simulink model "trial1"  (R2021a)
settings: Solver=VariableStepAuto  StartTime=0.0  StopTime=10  RelTol=1e-3
libraries: slpidlib x4, robotmobilelib x1
settings Model: Creator=templ  LastModifiedBy=templ

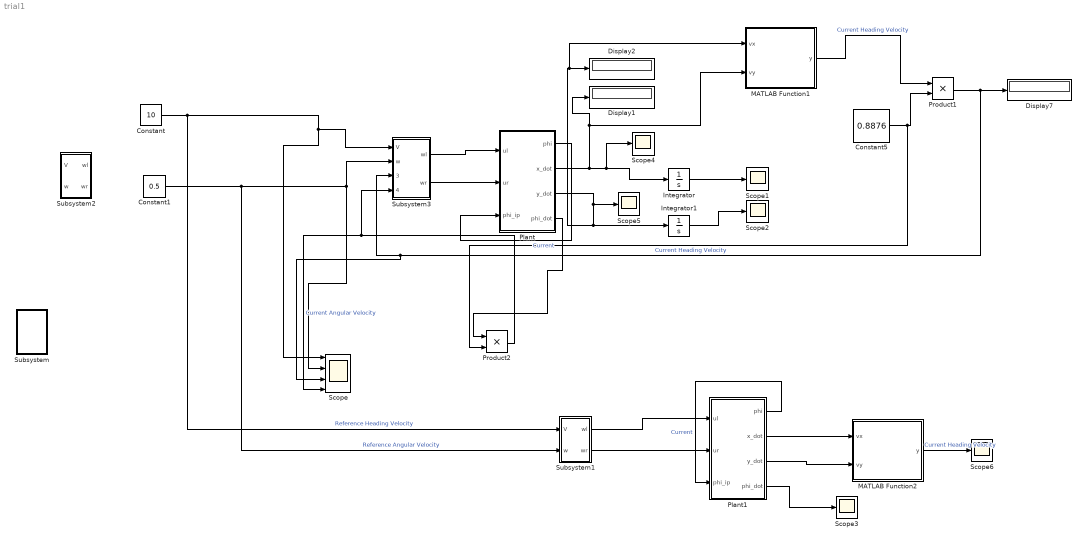
== system trial1 ==
  Constant : Constant  Value=10
  Constant1 : Constant  Value=0.5
  Constant5 : Constant  Value=0.8876
  Display1 : Display
  Display2 : Display
  Display7 : Display
  Integrator : Integrator
  Integrator1 : Integrator
  MATLAB Function1 : MATLAB Function  TreatAsAtomicUnit=on
  MATLAB Function2 : MATLAB Function  TreatAsAtomicUnit=on
  Plant : Subsystem
  Plant1 : Subsystem
  Product1 : Product
  Product2 : Product
  Scope : Scope  NumInputPorts=4
  Scope{1..6} (6 alike) : Scope
  Subsystem : Subsystem
  Subsystem1 : Subsystem
  Subsystem2 : Subsystem
  Subsystem3 : Subsystem
  wires:
  Plant/1(phi) -> Plant/3(phi_ip)  "Current"
  Plant/2(x_dot) -> MATLAB Function1/2(vy), Display1/1, Scope4/1, Integrator/1
  Plant/3(y_dot) -> Scope5/1, Integrator1/1, MATLAB Function1/1(vx), Display2/1
  Integrator/1 -> Scope1/1
  Integrator1/1 -> Scope2/1
  Plant/4(phi_dot) -> Product2/1
  MATLAB Function1/1(y) -> Product1/1  "Current Heading Velocity"
  Constant5/1 -> Product2/2, Product1/2
  Constant/1 -> Subsystem1/1(V), Scope/1, Subsystem3/1(V)  "Reference Heading Velocity"
  Constant1/1 -> Subsystem1/2(w), Subsystem3/2(w), Scope/2  "Reference Angular Velocity"
  Product1/1 -> Scope/3, Subsystem3/3(V_current), Display7/1  "Current Heading Velocity"
  Subsystem3/1(wl) -> Plant/1(ul)
  Subsystem3/2(wr) -> Plant/2(ur)
  Product2/1 -> Scope/4, Subsystem3/4(w_current)  "Current Angular Velocity"
  Plant1/1(phi) -> Plant1/3(phi_ip)  "Current"
  Plant1/2(x_dot) -> MATLAB Function2/1(vx)
  Plant1/3(y_dot) -> MATLAB Function2/2(vy)
  Plant1/4(phi_dot) -> Scope3/1
  MATLAB Function2/1(y) -> Scope6/1  "Current Heading Velocity"
  Subsystem1/1(wl) -> Plant1/1(ul)
  Subsystem1/2(wr) -> Plant1/2(ur)

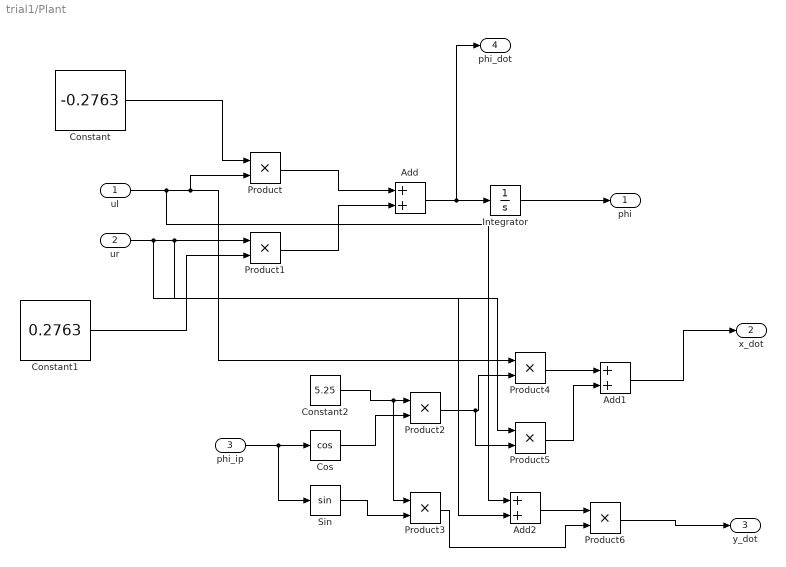
== system trial1/Plant ==
  ul : Inport
  ur : Inport  Port=2
  phi_ip : Inport  Port=3
  Add : Sum
  Add1 : Sum
  Add2 : Sum
  Constant : Constant  Value=-0.2763
  Constant1 : Constant  Value=0.2763
  Constant2 : Constant  Value=5.25
  Cos : Trigonometry  Operator=cos
  Integrator : Integrator
  Product{,1..6} (7 alike) : Product
  Sin : Trigonometry
  phi : Outport
  x_dot : Outport  Port=2
  y_dot : Outport  Port=3
  phi_dot : Outport  Port=4
  wires:
  ur/1 -> Add2/2, Product5/1, Product1/1
  Product/1 -> Add/1
  Integrator/1 -> phi/1
  Product1/1 -> Add/2
  Constant1/1 -> Product1/2
  Add/1 -> phi_dot/1, Integrator/1
  ul/1 -> Add2/1, Product4/1, Product/2
  Constant/1 -> Product/1
  phi_ip/1 -> Sin/1, Cos/1
  Cos/1 -> Product2/2
  Constant2/1 -> Product3/1, Product2/1
  Sin/1 -> Product3/2
  Product2/1 -> Product5/2, Product4/2
  Product4/1 -> Add1/1
  Product5/1 -> Add1/2
  Add1/1 -> x_dot/1
  Add2/1 -> Product6/1
  Product3/1 -> Product6/2
  Product6/1 -> y_dot/1

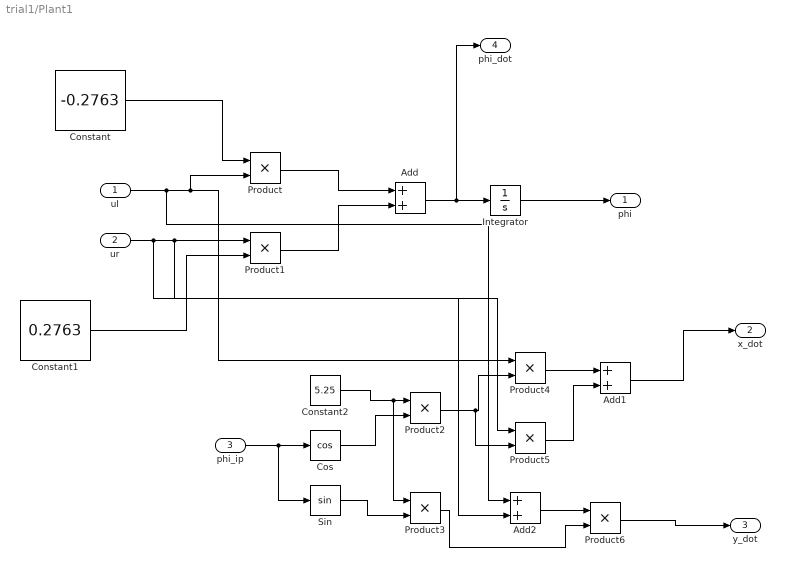
== system trial1/Plant1 ==
  ul : Inport
  ur : Inport  Port=2
  phi_ip : Inport  Port=3
  Add : Sum
  Add1 : Sum
  Add2 : Sum
  Constant : Constant  Value=-0.2763
  Constant1 : Constant  Value=0.2763
  Constant2 : Constant  Value=5.25
  Cos : Trigonometry  Operator=cos
  Integrator : Integrator
  Product{,1..6} (7 alike) : Product
  Sin : Trigonometry
  phi : Outport
  x_dot : Outport  Port=2
  y_dot : Outport  Port=3
  phi_dot : Outport  Port=4
  wires:
  ur/1 -> Add2/2, Product5/1, Product1/1
  Product/1 -> Add/1
  Integrator/1 -> phi/1
  Product1/1 -> Add/2
  Constant1/1 -> Product1/2
  Add/1 -> phi_dot/1, Integrator/1
  ul/1 -> Add2/1, Product4/1, Product/2
  Constant/1 -> Product/1
  phi_ip/1 -> Sin/1, Cos/1
  Cos/1 -> Product2/2
  Constant2/1 -> Product3/1, Product2/1
  Sin/1 -> Product3/2
  Product2/1 -> Product5/2, Product4/2
  Product4/1 -> Add1/1
  Product5/1 -> Add1/2
  Add1/1 -> x_dot/1
  Add2/1 -> Product6/1
  Product3/1 -> Product6/2
  Product6/1 -> y_dot/1

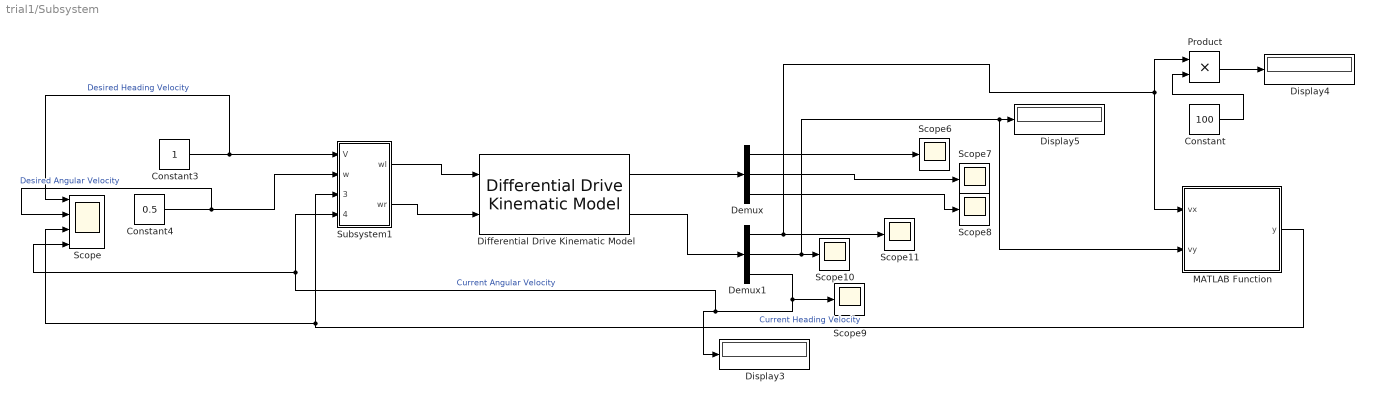
== system trial1/Subsystem ==
  Constant : Constant  Value=100
  Constant3 : Constant
  Constant4 : Constant  Value=0.5
  Demux : Demux  Outputs=3
  Demux1 : Demux  Outputs=3
  Differential Drive Kinematic Model : robotmobilelib/Differential Drive Kinematic Model  VehicleInputs=Wheel Speeds  WheelRadius=0.105  WheelSpeedRange=[-inf inf]  TrackWidth=0.05  InitialState=[0; 0; 0]  SimulateUsing=Interpreted execution
      settings: SourceProductBaseCode=RO
  Display3 : Display
  Display4 : Display
  Display5 : Display
  MATLAB Function : MATLAB Function  TreatAsAtomicUnit=on
  Product : Product
  Scope : Scope  NumInputPorts=4
  Scope{6..11} (6 alike) : Scope
  Subsystem1 : Subsystem
  wires:
  Demux1/2 -> MATLAB Function/2(vy), Display5/1, Scope10/1
  Differential Drive Kinematic Model/2 -> Demux1/1
  Constant3/1 -> Scope/1, Subsystem1/1(V)  "Desired Heading Velocity"
  MATLAB Function/1(y) -> Scope/3, Subsystem1/3(V_current)  "Current Heading Velocity"
  Demux1/1 -> MATLAB Function/1(vx), Product/1, Scope11/1
  Demux1/3 -> Scope/4, Subsystem1/4(w_current), Display3/1, Scope9/1  "Current Angular Velocity"
  Differential Drive Kinematic Model/1 -> Demux/1
  Demux/3 -> Scope8/1
  Constant4/1 -> Scope/2, Subsystem1/2(w)  "Desired Angular Velocity"
  Product/1 -> Display4/1
  Constant/1 -> Product/2
  Subsystem1/1(wl) -> Differential Drive Kinematic Model/1
  Subsystem1/2(wr) -> Differential Drive Kinematic Model/2
  Demux/2 -> Scope7/1
  Demux/1 -> Scope6/1

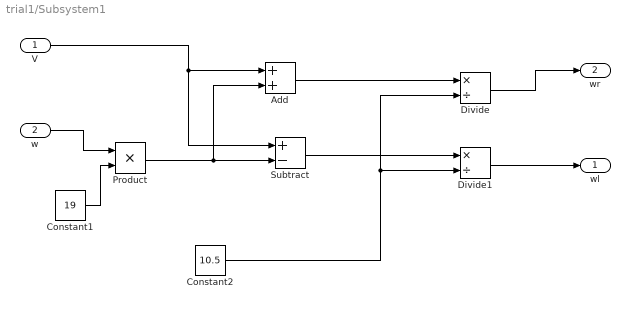
== system trial1/Subsystem1 ==
  V : Inport
  w : Inport  Port=2
  Add : Sum
  Constant1 : Constant  Value=19
  Constant2 : Constant  Value=10.5
  Divide : Product  Inputs=*/
  Divide1 : Product  Inputs=*/
  Product : Product
  Subtract : Sum  Inputs=+-
  wl : Outport
  wr : Outport  Port=2
  wires:
  V/1 -> Subtract/1, Add/1
  Add/1 -> Divide/1
  Constant2/1 -> Divide1/2, Divide/2
  Subtract/1 -> Divide1/1
  Product/1 -> Subtract/2, Add/2
  Divide1/1 -> wl/1
  Divide/1 -> wr/1
  Constant1/1 -> Product/2
  w/1 -> Product/1

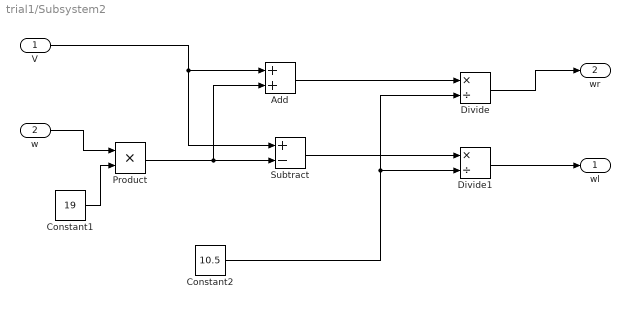
== system trial1/Subsystem2 ==
  V : Inport
  w : Inport  Port=2
  Add : Sum
  Constant1 : Constant  Value=19
  Constant2 : Constant  Value=10.5
  Divide : Product  Inputs=*/
  Divide1 : Product  Inputs=*/
  Product : Product
  Subtract : Sum  Inputs=+-
  wl : Outport
  wr : Outport  Port=2
  wires:
  V/1 -> Subtract/1, Add/1
  Add/1 -> Divide/1
  Constant2/1 -> Divide1/2, Divide/2
  Subtract/1 -> Divide1/1
  Product/1 -> Subtract/2, Add/2
  Divide1/1 -> wl/1
  Divide/1 -> wr/1
  Constant1/1 -> Product/2
  w/1 -> Product/1

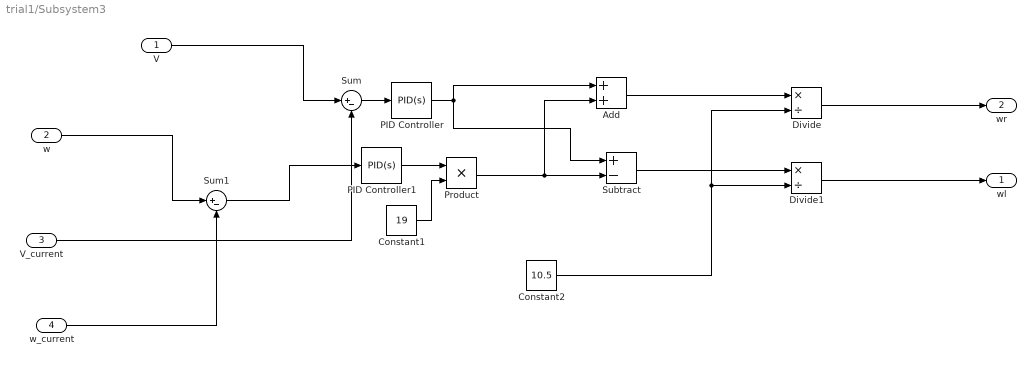
== system trial1/Subsystem3 ==
  V : Inport
  w : Inport  Port=2
  V_current : Inport  Port=3
  w_current : Inport  Port=4
  Add : Sum
  Constant1 : Constant  Value=19
  Constant2 : Constant  Value=10.5
  Divide : Product  Inputs=*/
  Divide1 : Product  Inputs=*/
  PID Controller : slpidlib/PID Controller  Controller=PID  Form=Parallel  TimeDomain=Continuous-time  UseExternalTs=off  SampleTime=-1  IntegratorMethod=Forward Euler  FilterMethod=Forward Euler  ControllerParametersSource=internal  P=10  I=1  D=5  UseFilter=on  N=100  TunerSelectOption=Transfer Function Based (PID Tuner App)  InitialConditionSource=internal  InitialConditionForIntegrator=0  InitialConditionForFilter=0  DifferentiatorICPrevScaledInput=0  ExternalReset=none  TrackingMode=off  Kt=1  LimitOutput=off  SatLimitsSource=internal  UpperSaturationLimit=inf  LowerSaturationLimit=-inf  LinearizeAsGain=on  AntiWindupMode=none  Kb=1  POutMin=[]  POutMax=[]  IOutMin=[]  IOutMax=[]  DOutMin=[]  DOutMax=[]  NOutMin=[]  NOutMax=[]  SumOutMin=[]  SumOutMax=[]  SaturationOutMin=[]  SaturationOutMax=[]  PParamMin=[]  PParamMax=[]  IParamMin=[]  IParamMax=[]  DParamMin=[]  DParamMax=[]  NParamMin=[]  NParamMax=[]  KbParamMin=[]  KbParamMax=[]  KtParamMin=[]  KtParamMax=[]  KbOutMin=[]  KbOutMax=[]  KtOutMin=[]  KtOutMax=[]  IntegratorOutMin=[]  IntegratorOutMax=[]  FilterOutMin=[]  FilterOutMax=[]  SumI1OutMin=[]  SumI1OutMax=[]  SumI2OutMin=[]  SumI2OutMax=[]  SumI3OutMin=[]  SumI3OutMax=[]  SumI4OutMin=[]  SumI4OutMax=[]  SumDOutMin=[]  SumDOutMax=[]  DifferentiatorOutMin=[]  DifferentiatorOutMax=[]  FilterDiffOutCoefMin=[]  FilterDiffOutCoefMax=[]  ReciprocalOutMin=[]  ReciprocalOutMax=[]  SumDenOutMin=[]  SumDenOutMax=[]  SumNumOutMin=[]  SumNumOutMax=[]  DivideOutMin=[]  DivideOutMax=[]  UdiffTsProdOutMin=[]  UdiffTsProdOutMax=[]  NTsProdOutMin=[]  NTsProdOutMax=[]  UintegralTsProdOutMin=[]  UintegralTsProdOutMax=[]  UngainTsProdOutMin=[]  UngainTsProdOutMax=[]  IntegratorContinuousStateAttributes=''  IntegratorStateMustResolveToSignalObject=off  IntegratorRTWStateStorageClass=Auto  FilterContinuousStateAttributes=''  FilterStateMustResolveToSignalObject=off  FilterRTWStateStorageClass=Auto  ParallelPVariant=InternalParameters  IdealPVariant=Disabled  IVariant=InternalParameters  DVariant=InternalParameters  IntegratorVariant=Continuous  SatVariant=Disabled  AWVariant=Passthrough  PCopyVariant=Disabled  TRVariant=Disabled  FdbkBlocksVariant=Forward  IdealPFdbkVariant=Disabled  SatFdbkVariant=Disabled  DerivativeFilterVariant=ContFilter  NVariant=InternalParameters  NCopyVariant=Disabled  FilterICVariant=InternalICsFilter  IntegratorICVariant=InternalICs  ExternalResetVariant=Disabled  TRSumVariant=Passthrough  SumFdbkVariant=Disabled  SumVariant=Sum_PID  TsampFilterVariant=InternalTs  TsampNgainVariant=Passthrough  TsampIntegralVariant=Passthrough  ExternalSaturationOutDataTypeStr=Inherit: Same as second input
  PID Controller1 : slpidlib/PID Controller  Controller=PID  Form=Parallel  TimeDomain=Continuous-time  UseExternalTs=off  SampleTime=-1  IntegratorMethod=Forward Euler  FilterMethod=Forward Euler  ControllerParametersSource=internal  P=10  I=1  D=5  UseFilter=on  N=100  TunerSelectOption=Transfer Function Based (PID Tuner App)  InitialConditionSource=internal  InitialConditionForIntegrator=0  InitialConditionForFilter=0  DifferentiatorICPrevScaledInput=0  ExternalReset=none  TrackingMode=off  Kt=1  LimitOutput=off  SatLimitsSource=internal  UpperSaturationLimit=inf  LowerSaturationLimit=-inf  LinearizeAsGain=on  AntiWindupMode=none  Kb=1  POutMin=[]  POutMax=[]  IOutMin=[]  IOutMax=[]  DOutMin=[]  DOutMax=[]  NOutMin=[]  NOutMax=[]  SumOutMin=[]  SumOutMax=[]  SaturationOutMin=[]  SaturationOutMax=[]  PParamMin=[]  PParamMax=[]  IParamMin=[]  IParamMax=[]  DParamMin=[]  DParamMax=[]  NParamMin=[]  NParamMax=[]  KbParamMin=[]  KbParamMax=[]  KtParamMin=[]  KtParamMax=[]  KbOutMin=[]  KbOutMax=[]  KtOutMin=[]  KtOutMax=[]  IntegratorOutMin=[]  IntegratorOutMax=[]  FilterOutMin=[]  FilterOutMax=[]  SumI1OutMin=[]  SumI1OutMax=[]  SumI2OutMin=[]  SumI2OutMax=[]  SumI3OutMin=[]  SumI3OutMax=[]  SumI4OutMin=[]  SumI4OutMax=[]  SumDOutMin=[]  SumDOutMax=[]  DifferentiatorOutMin=[]  DifferentiatorOutMax=[]  FilterDiffOutCoefMin=[]  FilterDiffOutCoefMax=[]  ReciprocalOutMin=[]  ReciprocalOutMax=[]  SumDenOutMin=[]  SumDenOutMax=[]  SumNumOutMin=[]  SumNumOutMax=[]  DivideOutMin=[]  DivideOutMax=[]  UdiffTsProdOutMin=[]  UdiffTsProdOutMax=[]  NTsProdOutMin=[]  NTsProdOutMax=[]  UintegralTsProdOutMin=[]  UintegralTsProdOutMax=[]  UngainTsProdOutMin=[]  UngainTsProdOutMax=[]  IntegratorContinuousStateAttributes=''  IntegratorStateMustResolveToSignalObject=off  IntegratorRTWStateStorageClass=Auto  FilterContinuousStateAttributes=''  FilterStateMustResolveToSignalObject=off  FilterRTWStateStorageClass=Auto  ParallelPVariant=InternalParameters  IdealPVariant=Disabled  IVariant=InternalParameters  DVariant=InternalParameters  IntegratorVariant=Continuous  SatVariant=Disabled  AWVariant=Passthrough  PCopyVariant=Disabled  TRVariant=Disabled  FdbkBlocksVariant=Forward  IdealPFdbkVariant=Disabled  SatFdbkVariant=Disabled  DerivativeFilterVariant=ContFilter  NVariant=InternalParameters  NCopyVariant=Disabled  FilterICVariant=InternalICsFilter  IntegratorICVariant=InternalICs  ExternalResetVariant=Disabled  TRSumVariant=Passthrough  SumFdbkVariant=Disabled  SumVariant=Sum_PID  TsampFilterVariant=InternalTs  TsampNgainVariant=Passthrough  TsampIntegralVariant=Passthrough  ExternalSaturationOutDataTypeStr=Inherit: Same as second input
  Product : Product
  Subtract : Sum  Inputs=+-
  Sum : Sum  Inputs=|+-
  Sum1 : Sum  Inputs=|+-
  wl : Outport
  wr : Outport  Port=2
  wires:
  V/1 -> Sum/1
  Add/1 -> Divide/1
  Constant2/1 -> Divide1/2, Divide/2
  Subtract/1 -> Divide1/1
  Product/1 -> Subtract/2, Add/2
  Constant1/1 -> Product/2
  w/1 -> Sum1/1
  V_current/1 -> Sum/2
  Sum/1 -> PID Controller/1
  w_current/1 -> Sum1/2
  Sum1/1 -> PID Controller1/1
  PID Controller/1 -> Subtract/1, Add/1
  PID Controller1/1 -> Product/1
  Divide/1 -> wr/1
  Divide1/1 -> wl/1

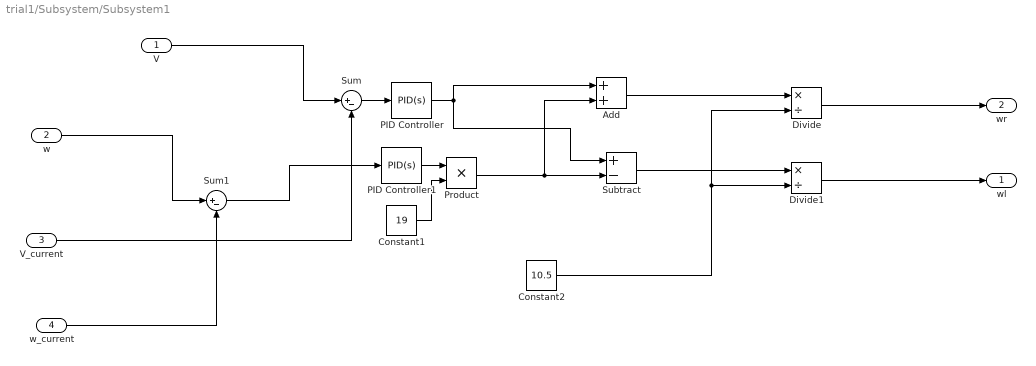
== system trial1/Subsystem/Subsystem1 ==
  V : Inport
  w : Inport  Port=2
  V_current : Inport  Port=3
  w_current : Inport  Port=4
  Add : Sum
  Constant1 : Constant  Value=19
  Constant2 : Constant  Value=10.5
  Divide : Product  Inputs=*/
  Divide1 : Product  Inputs=*/
  PID Controller : slpidlib/PID Controller  Controller=PID  Form=Parallel  TimeDomain=Continuous-time  UseExternalTs=off  SampleTime=-1  IntegratorMethod=Forward Euler  FilterMethod=Forward Euler  ControllerParametersSource=internal  P=-500  I=100  D=1  UseFilter=on  N=100  TunerSelectOption=Frequency Response Based  InitialConditionSource=internal  InitialConditionForIntegrator=0  InitialConditionForFilter=0  DifferentiatorICPrevScaledInput=0  ExternalReset=none  TrackingMode=off  Kt=1  LimitOutput=off  SatLimitsSource=internal  UpperSaturationLimit=inf  LowerSaturationLimit=-inf  LinearizeAsGain=on  AntiWindupMode=none  Kb=1  POutMin=[]  POutMax=[]  IOutMin=[]  IOutMax=[]  DOutMin=[]  DOutMax=[]  NOutMin=[]  NOutMax=[]  SumOutMin=[]  SumOutMax=[]  SaturationOutMin=[]  SaturationOutMax=[]  PParamMin=[]  PParamMax=[]  IParamMin=[]  IParamMax=[]  DParamMin=[]  DParamMax=[]  NParamMin=[]  NParamMax=[]  KbParamMin=[]  KbParamMax=[]  KtParamMin=[]  KtParamMax=[]  KbOutMin=[]  KbOutMax=[]  KtOutMin=[]  KtOutMax=[]  IntegratorOutMin=[]  IntegratorOutMax=[]  FilterOutMin=[]  FilterOutMax=[]  SumI1OutMin=[]  SumI1OutMax=[]  SumI2OutMin=[]  SumI2OutMax=[]  SumI3OutMin=[]  SumI3OutMax=[]  SumI4OutMin=[]  SumI4OutMax=[]  SumDOutMin=[]  SumDOutMax=[]  DifferentiatorOutMin=[]  DifferentiatorOutMax=[]  FilterDiffOutCoefMin=[]  FilterDiffOutCoefMax=[]  ReciprocalOutMin=[]  ReciprocalOutMax=[]  SumDenOutMin=[]  SumDenOutMax=[]  SumNumOutMin=[]  SumNumOutMax=[]  DivideOutMin=[]  DivideOutMax=[]  UdiffTsProdOutMin=[]  UdiffTsProdOutMax=[]  NTsProdOutMin=[]  NTsProdOutMax=[]  UintegralTsProdOutMin=[]  UintegralTsProdOutMax=[]  UngainTsProdOutMin=[]  UngainTsProdOutMax=[]  IntegratorContinuousStateAttributes=''  IntegratorStateMustResolveToSignalObject=off  IntegratorRTWStateStorageClass=Auto  FilterContinuousStateAttributes=''  FilterStateMustResolveToSignalObject=off  FilterRTWStateStorageClass=Auto  ParallelPVariant=InternalParameters  IdealPVariant=Disabled  IVariant=InternalParameters  DVariant=InternalParameters  IntegratorVariant=Continuous  SatVariant=Disabled  AWVariant=Passthrough  PCopyVariant=Disabled  TRVariant=Disabled  FdbkBlocksVariant=Forward  IdealPFdbkVariant=Disabled  SatFdbkVariant=Disabled  DerivativeFilterVariant=ContFilter  NVariant=InternalParameters  NCopyVariant=Disabled  FilterICVariant=InternalICsFilter  IntegratorICVariant=InternalICs  ExternalResetVariant=Disabled  TRSumVariant=Passthrough  SumFdbkVariant=Disabled  SumVariant=Sum_PID  TsampFilterVariant=InternalTs  TsampNgainVariant=Passthrough  TsampIntegralVariant=Passthrough  ExternalSaturationOutDataTypeStr=Inherit: Same as second input
  PID Controller1 : slpidlib/PID Controller  Controller=PID  Form=Parallel  TimeDomain=Continuous-time  UseExternalTs=off  SampleTime=-1  IntegratorMethod=Forward Euler  FilterMethod=Forward Euler  ControllerParametersSource=internal  P=-500  I=100  D=1  UseFilter=on  N=100  TunerSelectOption=Transfer Function Based (PID Tuner App)  InitialConditionSource=internal  InitialConditionForIntegrator=0  InitialConditionForFilter=0  DifferentiatorICPrevScaledInput=0  ExternalReset=none  TrackingMode=off  Kt=1  LimitOutput=off  SatLimitsSource=internal  UpperSaturationLimit=inf  LowerSaturationLimit=-inf  LinearizeAsGain=on  AntiWindupMode=none  Kb=1  POutMin=[]  POutMax=[]  IOutMin=[]  IOutMax=[]  DOutMin=[]  DOutMax=[]  NOutMin=[]  NOutMax=[]  SumOutMin=[]  SumOutMax=[]  SaturationOutMin=[]  SaturationOutMax=[]  PParamMin=[]  PParamMax=[]  IParamMin=[]  IParamMax=[]  DParamMin=[]  DParamMax=[]  NParamMin=[]  NParamMax=[]  KbParamMin=[]  KbParamMax=[]  KtParamMin=[]  KtParamMax=[]  KbOutMin=[]  KbOutMax=[]  KtOutMin=[]  KtOutMax=[]  IntegratorOutMin=[]  IntegratorOutMax=[]  FilterOutMin=[]  FilterOutMax=[]  SumI1OutMin=[]  SumI1OutMax=[]  SumI2OutMin=[]  SumI2OutMax=[]  SumI3OutMin=[]  SumI3OutMax=[]  SumI4OutMin=[]  SumI4OutMax=[]  SumDOutMin=[]  SumDOutMax=[]  DifferentiatorOutMin=[]  DifferentiatorOutMax=[]  FilterDiffOutCoefMin=[]  FilterDiffOutCoefMax=[]  ReciprocalOutMin=[]  ReciprocalOutMax=[]  SumDenOutMin=[]  SumDenOutMax=[]  SumNumOutMin=[]  SumNumOutMax=[]  DivideOutMin=[]  DivideOutMax=[]  UdiffTsProdOutMin=[]  UdiffTsProdOutMax=[]  NTsProdOutMin=[]  NTsProdOutMax=[]  UintegralTsProdOutMin=[]  UintegralTsProdOutMax=[]  UngainTsProdOutMin=[]  UngainTsProdOutMax=[]  IntegratorContinuousStateAttributes=''  IntegratorStateMustResolveToSignalObject=off  IntegratorRTWStateStorageClass=Auto  FilterContinuousStateAttributes=''  FilterStateMustResolveToSignalObject=off  FilterRTWStateStorageClass=Auto  ParallelPVariant=InternalParameters  IdealPVariant=Disabled  IVariant=InternalParameters  DVariant=InternalParameters  IntegratorVariant=Continuous  SatVariant=Disabled  AWVariant=Passthrough  PCopyVariant=Disabled  TRVariant=Disabled  FdbkBlocksVariant=Forward  IdealPFdbkVariant=Disabled  SatFdbkVariant=Disabled  DerivativeFilterVariant=ContFilter  NVariant=InternalParameters  NCopyVariant=Disabled  FilterICVariant=InternalICsFilter  IntegratorICVariant=InternalICs  ExternalResetVariant=Disabled  TRSumVariant=Passthrough  SumFdbkVariant=Disabled  SumVariant=Sum_PID  TsampFilterVariant=InternalTs  TsampNgainVariant=Passthrough  TsampIntegralVariant=Passthrough  ExternalSaturationOutDataTypeStr=Inherit: Same as second input
  Product : Product
  Subtract : Sum  Inputs=+-
  Sum : Sum  Inputs=|+-
  Sum1 : Sum  Inputs=|+-
  wl : Outport
  wr : Outport  Port=2
  wires:
  V/1 -> Sum/1
  Add/1 -> Divide/1
  Constant2/1 -> Divide1/2, Divide/2
  Subtract/1 -> Divide1/1
  Product/1 -> Subtract/2, Add/2
  Divide1/1 -> wl/1
  Divide/1 -> wr/1
  Constant1/1 -> Product/2
  w/1 -> Sum1/1
  V_current/1 -> Sum/2
  Sum/1 -> PID Controller/1
  w_current/1 -> Sum1/2
  Sum1/1 -> PID Controller1/1
  PID Controller/1 -> Subtract/1, Add/1
  PID Controller1/1 -> Product/1

== matlab function trial1/Subsystem/MATLAB Function ==
  data: vx input; y output; vy input
function y = fcn(vx,vy)
vnet=sqrt((vx^2)+(vy^2));



y = vnet;

== matlab function trial1/MATLAB Function2 ==
  data: vx input; y output; vy input
function y = fcn(vx,vy)
vnet=sqrt((vx^2)+(vy^2));



y = vnet;

== matlab function trial1/MATLAB Function1 ==
  data: vx input; y output; vy input
function y = fcn(vx,vy)
vnet=sqrt((vx^2)+(vy^2));



y = vnet;
